simulink model "passivity_based_control"  (R2025a)
settings: Solver=VariableStepAuto  StartTime=0.0  StopTime=115  RelTol=1e-3
values from neighbouring files (symbols this model uses):
  Dxy = 1    [main_passivity_based_control.m]
  Dyaw = -0.8    [main_passivity_based_control.m]
  eta_b_0 = [0 0 0]    [main_passivity_based_control.m]
  eta_b_dot_0 = [0 0 0]    [main_passivity_based_control.m]
  f_e = [Dxy Dxy Dz]    [main_passivity_based_control.m]
  g = 9.81    [main_passivity_based_control.m]
  Ib = diag([1.2416 1.2416 2*1.2416])    [main_passivity_based_control.m]
  K = flip(K)    [main_passivity_based_control.m]
  K_a = 1.25    [main_passivity_based_control.m]
  K_r = 0.5    [main_passivity_based_control.m]
  lin_vel_0 = [0; 0; 0]    [main_passivity_based_control.m]
  mass = 1.2    [main_passivity_based_control.m]
  obstacles_points = [obstacles_points, points]    [main_passivity_based_control.m]
  pos_0 = [x0 y0 z0]    [main_passivity_based_control.m]
  psif = 0    [main_passivity_based_control.m]
  r = 2    [main_passivity_based_control.m]
  rho_0 = 2.0    (= 2)    [main_passivity_based_control.m]
  tau_e = [0 0 Dyaw]    [main_passivity_based_control.m]
  Ts = 0.01    [main_passivity_based_control.m]
  Waypoints = [ 0  20  -6 ... (first row only)    [main_passivity_based_control.m]
undefined symbols (not defined in the file or in its folder): DiscIntNeverNeededParam
libraries: uavsimlib x3, robotcorelib x1, eeGeneralControl x1
settings Model: Creator=emman  LastModifiedBy=emman

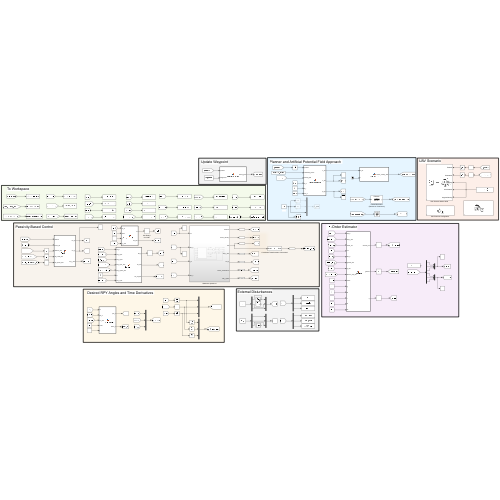
[thumbnail: Simulink's stored preview of the top-level diagram]
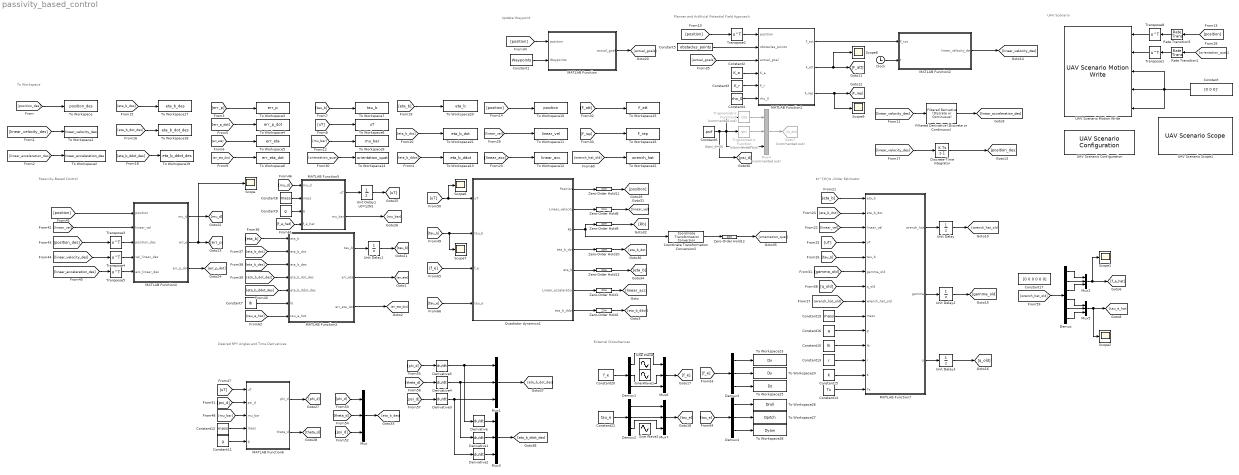
== system passivity_based_control ==
  note: Passivity-Based Control
  note: Desired RPY Angles and Time Derivatives
  note: Update Waypoint
  note: Planner and Artificial Potential Field Approach
  note: UAV Scenario
  note: $\psi_d=0$
  note: To Workspace
  note: $r^{th}$ -Order Estimator
  note: External Disturbances
  Clock : Clock
  Constant : Constant  Value=[0 0 0]'
  Constant1 : Constant  Value=Waypoints
  Constant10 : Constant  Value=Ib
  Constant11 : Constant  Value=g
  Constant12 : Constant  Value=mass
  Constant13 : Constant  Value=r
  Constant14 : Constant  Value=Ts
  Constant15 : Constant  Value=K
  Constant16 : Constant  Value=g
  Constant17 : Constant  Value=[0 0 0 0 0 0]
  Constant19 : Constant  Value=mass
  Constant2 : Constant  Value=K_a
  Constant20 : Constant  Value=f_e
  Constant21 : Constant  Value=tau_e
  Constant3 : Constant  Value=K_r
  Constant4 : Constant  Value=rho_0
  Constant5 : Constant  Value=obstacles_points
  Constant6 : Constant  Value=psif
  Constant7 : Constant  Value=Ib
  Constant8 : Constant  Value=mass
  Constant9 : Constant  Value=g
  Coordinate Transformation Conversion2 : robotcorelib/Coordinate Transformation Conversion  InputRepresentation=Rotation Matrix  InputEulerSequence=ZYX  ShowTrVecInputPort=on  OutputRepresentation=Quaternion  OutputEulerSequence=ZYX  ShowTrVecOutputPort=on  SimulateUsing=Interpreted execution
  Demux : Demux  Outputs=6
  Demux{1..4} (4 alike) : Demux  Outputs=3
  Derivative{,1..5} (6 alike) : Derivative
  Discrete-Time Integrator : DiscreteIntegrator  InitialCondition=pos_0  SampleTime=Ts  ICPrevOutput=DiscIntNeverNeededParam  ICPrevScaledInput=DiscIntNeverNeededParam
  Filtered Derivative (Discrete or Continuous) : eeGeneralControl/Filtered Derivative (Discrete or Continuous)  K=1  T=Ts  B=inf  A=-inf  minRatio=10  init_option=Inherited from block input  x0=0  Ts=-1
      settings: LibrarySourceBlock=|
      | ee_sl_lib/General Control/Filtered Derivative
      | (Discrete or Continuous)
  Goto7 : Goto  Commented=on  GotoTag=xb_des
  MATLAB Function : MATLAB Function  TreatAsAtomicUnit=on
  MATLAB Function1 : MATLAB Function  TreatAsAtomicUnit=on
  MATLAB Function2 : MATLAB Function  TreatAsAtomicUnit=on
  MATLAB Function3 : MATLAB Function  TreatAsAtomicUnit=on
  MATLAB Function4 : MATLAB Function  TreatAsAtomicUnit=on
  MATLAB Function5 : MATLAB Function  TreatAsAtomicUnit=on
  MATLAB Function6 : MATLAB Function  TreatAsAtomicUnit=on
  MATLAB Function7 : MATLAB Function  TreatAsAtomicUnit=on
  Mux{,1..3,5..7} (7 alike) : Mux  Inputs=3
  Mux4 : Mux  Commented=on  Inputs=3
  Quadrotor dynamics1 : Subsystem
  Rate Transition1 : RateTransition  OutPortSampleTime=Ts
  Rate Transition5 : RateTransition  OutPortSampleTime=Ts
  Scope{,1..2,6..9} (7 alike) : Scope
      Scope settings: ActiveDisplayYMinimum=-1  ActiveDisplayYMaximum=1  DataLoggingVariableName=ScopeData3
      Scope1 settings: ActiveDisplayYMinimum=-1  ActiveDisplayYMaximum=1
      Scope2 settings: ActiveDisplayYMinimum=-2.2549630226203039  ActiveDisplayYMaximum=1.6732320406118144
      Scope6 settings: ActiveDisplayYMinimum=11.66748  ActiveDisplayYMaximum=12.03695  DataLoggingVariableName=ScopeData2
      Scope7 settings: ActiveDisplayYMinimum=-0.02035  ActiveDisplayYMaximum=0.02035  DataLoggingVariableName=ScopeData7
      Scope8 settings: ActiveDisplayYMinimum=-10.489441161556352  ActiveDisplayYMaximum=10.433654100091561  DataLoggingVariableName=ScopeData8
      Scope9 settings: ActiveDisplayYMinimum=-1  ActiveDisplayYMaximum=1  DataLoggingVariableName=ScopeData9
  Sine Wave : Sin  Amplitude=Dxy  Frequency=0.5  SampleTime=Ts
  Sine Wave1 : Sin  Amplitude=Dxy  Frequency=0.2  Phase=pi  SampleTime=Ts
  Sine Wave2 : Sin  Amplitude=Dyaw  Frequency=0.1  SampleTime=Ts
  To Workspace : ToWorkspace  VariableName=position_des  SaveFormat=Timeseries  SampleTime=-1
  To Workspace1 : ToWorkspace  VariableName=linear_velocity_des  SaveFormat=Timeseries  SampleTime=-1
  To Workspace10 : ToWorkspace  VariableName=position  SaveFormat=Timeseries  SampleTime=-1
  To Workspace11 : ToWorkspace  VariableName=linear_vel  SaveFormat=Timeseries  SampleTime=-1
  To Workspace12 : ToWorkspace  VariableName=linear_acc  SaveFormat=Timeseries  SampleTime=-1
  To Workspace13 : ToWorkspace  VariableName=eta_b_ddot  SaveFormat=Timeseries  SampleTime=-1
  To Workspace14 : ToWorkspace  VariableName=orientation_quat  SaveFormat=Timeseries  SampleTime=-1
  To Workspace15 : ToWorkspace  VariableName=F_att  SaveFormat=Timeseries  SampleTime=-1
  To Workspace16 : ToWorkspace  VariableName=F_rep  SaveFormat=Timeseries  SampleTime=-1
  To Workspace17 : ToWorkspace  VariableName=eta_b_des  SaveFormat=Timeseries  SampleTime=-1
  To Workspace18 : ToWorkspace  VariableName=eta_b_dot_des  SaveFormat=Timeseries  SampleTime=-1
  To Workspace19 : ToWorkspace  VariableName=eta_b_ddot_des  SaveFormat=Timeseries  SampleTime=-1
  To Workspace2 : ToWorkspace  VariableName=linear_acceleration_des  SaveFormat=Timeseries  SampleTime=-1
  To Workspace20 : ToWorkspace  VariableName=eta_b  SaveFormat=Timeseries  SampleTime=-1
  To Workspace21 : ToWorkspace  VariableName=eta_b_dot  SaveFormat=Timeseries  SampleTime=-1
  To Workspace22 : ToWorkspace  VariableName=wrench_hat  SaveFormat=Timeseries  SampleTime=-1
  To Workspace23 : ToWorkspace  VariableName=Dx  SaveFormat=Timeseries  SampleTime=-1
  To Workspace24 : ToWorkspace  VariableName=Dy  SaveFormat=Timeseries  SampleTime=-1
  To Workspace25 : ToWorkspace  VariableName=Dz  SaveFormat=Timeseries  SampleTime=-1
  To Workspace26 : ToWorkspace  VariableName=Droll  SaveFormat=Timeseries  SampleTime=-1
  To Workspace27 : ToWorkspace  VariableName=Dpitch  SaveFormat=Timeseries  SampleTime=-1
  To Workspace28 : ToWorkspace  VariableName=Dyaw  SaveFormat=Timeseries  SampleTime=-1
  To Workspace3 : ToWorkspace  VariableName=err_p  SaveFormat=Timeseries  SampleTime=-1
  To Workspace4 : ToWorkspace  VariableName=err_p_dot  SaveFormat=Timeseries  SampleTime=-1
  To Workspace5 : ToWorkspace  VariableName=err_eta  SaveFormat=Timeseries  SampleTime=-1
  To Workspace6 : ToWorkspace  VariableName=err_eta_dot  SaveFormat=Timeseries  SampleTime=-1
  To Workspace7 : ToWorkspace  VariableName=tau_b  SaveFormat=Timeseries  SampleTime=-1
  To Workspace8 : ToWorkspace  VariableName=uT  SaveFormat=Timeseries  SampleTime=-1
  To Workspace9 : ToWorkspace  VariableName=mu_bar  SaveFormat=Timeseries  SampleTime=-1
  Transpose{1..5,8} (6 alike) : Math  Operator=transpose
  Trigonometric Function : Trigonometry  Commented=on
  Trigonometric Function1 : Trigonometry  Commented=on  Operator=cos
  UAV Scenario Configuration : uavsimlib/UAV Scenario Configuration  Priority=-1  UAVScenarioObject=Scenario  SampleTime=Ts  UpdateParam=false  SensorMotionBusName='SensorMotionBus'  PlatformMotionBusName='PlatformMotionBus'  ScenarioMotionBusName='ScenarioMotionBus'  ScenarioMotionSignalName='ScenarioMotions'
  UAV Scenario Motion Write : uavsimlib/UAV Scenario Motion Write  Priority=0  PlatName='UAV'  ReferenceFrame=NED
  UAV Scenario Scope1 : uavsimlib/UAV Scenario Scope  Priority=1  SensorNameTable={}  SampleTime=Ts
  Unit Delay : UnitDelay  InitialCondition=zeros(6,1)  SampleTime=Ts  HasFrameUpgradeWarning=on
  Unit Delay1 : UnitDelay  InitialCondition=[0 0 0]'  SampleTime=Ts
  Unit Delay1 u0=12N1 : UnitDelay  InitialCondition=12  SampleTime=Ts
  Unit Delay2 : UnitDelay  InitialCondition=zeros(6,r)  SampleTime=Ts  HasFrameUpgradeWarning=on
  Unit Delay3 : UnitDelay  InitialCondition=zeros(6,1)  SampleTime=Ts  HasFrameUpgradeWarning=on
  Zero-Order Hold{1..2,8..13} (8 alike) : ZeroOrderHold  SampleTime=Ts
  wires:
  [linear_velocity_des] -> To Workspace1/1
  [tau_b] -> To Workspace7/1
  [err_eta] -> To Workspace5/1
  [position_des] -> To Workspace/1
  [linear_acceleration_des] -> To Workspace2/1
  [uT] -> To Workspace8/1
  [mu_bar] -> To Workspace9/1
  [err_p] -> To Workspace3/1
  Constant2/1 -> MATLAB Function1/4(K_a)
  Constant3/1 -> MATLAB Function1/5(K_r)
  Constant4/1 -> MATLAB Function1/6(rho_0)
  MATLAB Function1/1(F_tot) -> MATLAB Function2/1(F_tot)
  Clock/1 -> MATLAB Function2/2(t)
  MATLAB Function1/2(F_att) -> Scope8/1, [F_att]
  Trigonometric Function1/1 -> Mux4/1
  Mux4/1 -> Goto7/1
  Constant6/1 -> [psi_d], Mux4/3, Trigonometric Function/1, Trigonometric Function1/1
  Trigonometric Function/1 -> Mux4/2
  [linear_velocity_des] -> Filtered Derivative (Discrete or Continuous)/1
  [linear_velocity_des] -> Discrete-Time Integrator/1
  Constant/1 -> UAV Scenario Motion Write/5, UAV Scenario Motion Write/3, UAV Scenario Motion Write/4
  Constant5/1 -> MATLAB Function1/2(obstacles_points)
  Rate Transition5/1 -> Transpose8/1
  [position] -> Rate Transition5/1
  Transpose8/1 -> UAV Scenario Motion Write/1
  Rate Transition1/1 -> Transpose1/1
  Transpose1/1 -> UAV Scenario Motion Write/2
  [orientation_quat] -> Rate Transition1/1
  [position] -> To Workspace10/1
  [linear_acc] -> To Workspace12/1
  [linear_vel] -> To Workspace11/1
  [eta_b_ddot] -> To Workspace13/1
  [orientation_quat] -> To Workspace14/1
  [F_rep] -> To Workspace16/1
  [F_att] -> To Workspace15/1
  [position] -> Transpose2/1
  Transpose2/1 -> MATLAB Function1/1(position)
  MATLAB Function1/3(F_rep) -> [F_rep], Scope9/1
  [actual_goals] -> MATLAB Function1/3(actual_goal)
  Constant1/1 -> MATLAB Function/2(Waypoints)
  MATLAB Function/1(actual_goal) -> [actual_goals]
  [position] -> MATLAB Function/1(position)
  [eta_b] -> MATLAB Function3/1(eta_b)
  [eta_b_dot] -> MATLAB Function3/2(eta_b_dot)
  [eta_b_des] -> MATLAB Function3/3(eta_b_des)
  [eta_b_dot_des] -> MATLAB Function3/4(eta_b_dot_des)
  [eta_b_ddot_des] -> MATLAB Function3/5(eta_b_ddot_des)
  Constant7/1 -> MATLAB Function3/6(Ib)
  MATLAB Function3/1(tau_b) -> Unit Delay1/1
  Unit Delay1/1 -> [tau_b]
  [linear_acceleration_des] -> Transpose5/1
  [linear_velocity_des] -> Transpose4/1
  [position_des] -> Transpose3/1
  [linear_vel] -> MATLAB Function4/2(linear_vel)
  [position] -> MATLAB Function4/1(position)
  MATLAB Function4/1(mu_d) -> [mu_d]
  MATLAB Function4/3(err_p_dot) -> [err_p_dot]
  MATLAB Function4/2(err_p) -> Scope/1, [err_p]
  Constant9/1 -> MATLAB Function5/3(g)
  Constant8/1 -> MATLAB Function5/2(mass)
  [mu_d] -> MATLAB Function5/1(mu_d)
  MATLAB Function5/1(uT) -> Unit Delay1 u0=12N1/1
  Unit Delay1 u0=12N1/1 -> [uT]
  MATLAB Function5/2(mu_bar) -> [mu_bar]
  [uT] -> MATLAB Function6/1(uT)
  [mu_bar] -> MATLAB Function6/3(mu_bar)
  Constant12/1 -> MATLAB Function6/4(mass)
  Constant11/1 -> MATLAB Function6/5(g)
  MATLAB Function6/1(phi_d) -> [phi_d]
  MATLAB Function6/2(theta_d) -> [theta_d]
  Quadrotor dynamics1/3(Rb) -> Zero-Order Hold9/1, Coordinate Transformation Conversion2/1
  [tau_b] -> Quadrotor dynamics1/2(tau_b), Scope7/1
  Zero-Order Hold11/1 -> [position]
  Zero-Order Hold12/1 -> [orientation_quat]
  Zero-Order Hold8/1 -> [linear_vel]
  Coordinate Transformation Conversion2/1 -> Zero-Order Hold12/1
  Quadrotor dynamics1/1(Position) -> Zero-Order Hold11/1
  [uT] -> Scope6/1, Quadrotor dynamics1/1(uT)
  Quadrotor dynamics1/2(Linear_velocity) -> Zero-Order Hold8/1
  Zero-Order Hold9/1 -> [Rb]
  Quadrotor dynamics1/4(eta_b_dot) -> Zero-Order Hold10/1
  Quadrotor dynamics1/5(eta_b) -> Zero-Order Hold13/1
  [psi_d] -> MATLAB Function6/2(psi_d)
  [phi_d] -> Mux/1
  [theta_d] -> Mux/2
  [psi_d] -> Mux/3
  Mux/1 -> [eta_b_des]
  [phi_d] -> Derivative5/1
  [theta_d] -> Derivative4/1
  [psi_d] -> Derivative3/1
  Derivative3/1 -> Derivative2/1, Mux1/3
  Derivative4/1 -> Derivative1/1, Mux1/2
  Derivative5/1 -> Derivative/1, Mux1/1
  Mux1/1 -> [eta_b_dot_des]
  Derivative1/1 -> Mux3/2
  Derivative2/1 -> Mux3/3
  Derivative/1 -> Mux3/1
  Mux3/1 -> [eta_b_ddot_des]
  Transpose3/1 -> MATLAB Function4/3(position_des)
  Transpose4/1 -> MATLAB Function4/4(vel_linear_des)
  Transpose5/1 -> MATLAB Function4/5(acc_linear_des)
  MATLAB Function2/1(linear_velocity_des) -> [linear_velocity_des]
  Discrete-Time Integrator/1 -> [position_des]
  Zero-Order Hold10/1 -> [eta_b_dot]
  Zero-Order Hold13/1 -> [eta_b]
  Filtered Derivative (Discrete or Continuous)/1 -> [linear_acceleration_des]
  MATLAB Function3/3(err_eta_dot) -> [err_eta_dot]
  MATLAB Function3/2(err_eta) -> [err_eta]
  Quadrotor dynamics1/6(Linear_acceleration) -> Zero-Order Hold1/1
  Zero-Order Hold1/1 -> [linear_acc]
  Quadrotor dynamics1/7(eta_b_ddot) -> Zero-Order Hold2/1
  Zero-Order Hold2/1 -> [eta_b_ddot]
  [err_p_dot] -> To Workspace4/1
  [err_eta_dot] -> To Workspace6/1
  [eta_b_des] -> To Workspace17/1
  [eta_b_dot_des] -> To Workspace18/1
  [eta_b_ddot_des] -> To Workspace19/1
  [eta_b] -> To Workspace20/1
  [eta_b_dot] -> To Workspace21/1
  [q_old] -> MATLAB Function7/7(q_old)
  [wrench_hat_old] -> MATLAB Function7/8(wrench_hat_old)
  Demux/4 -> Mux5/1
  Demux/5 -> Mux5/2
  Mux2/1 -> Scope1/1, [f_e_hat]
  Demux/6 -> Mux5/3
  [gamma_old] -> MATLAB Function7/6(gamma_old)
  Demux/1 -> Mux2/1
  Unit Delay2/1 -> [gamma_old]
  Demux/2 -> Mux2/2
  MATLAB Function7/3(q) -> Unit Delay3/1
  MATLAB Function7/1(wrench_hat) -> Unit Delay/1
  Constant10/1 -> MATLAB Function7/11(Ib)
  [tau_b] -> MATLAB Function7/5(tau_b)
  [linear_vel] -> MATLAB Function7/3(linear_vel)
  Mux5/1 -> Scope2/1, [tau_e_hat]
  Unit Delay/1 -> [wrench_hat_old]
  MATLAB Function7/2(gamma) -> Unit Delay2/1
  [uT] -> MATLAB Function7/4(uT)
  Constant13/1 -> MATLAB Function7/12(r)
  Constant14/1 -> MATLAB Function7/14(Ts)
  Constant16/1 -> MATLAB Function7/10(g)
  Demux/3 -> Mux2/3
  Constant19/1 -> MATLAB Function7/9(mass)
  Unit Delay3/1 -> [q_old]
  Constant15/1 -> MATLAB Function7/13(K)
  [eta_b] -> MATLAB Function7/1(eta_b)
  [eta_b_dot] -> MATLAB Function7/2(eta_b_dot)
  [wrench_hat_old] -> To Workspace22/1
  [f_e_hat] -> MATLAB Function5/4(f_e_hat)
  [tau_e_hat] -> MATLAB Function3/7(tau_e_hat)
  [f_e] -> Quadrotor dynamics1/3(f_e)
  [tau_e] -> Quadrotor dynamics1/4(tau_e)
  Demux4/2 -> To Workspace27/1
  Demux4/3 -> To Workspace28/1
  Demux3/1 -> To Workspace23/1
  [tau_e] -> Demux4/1
  Demux3/3 -> To Workspace25/1
  [f_e] -> Demux3/1
  Demux4/1 -> To Workspace26/1
  Mux7/1 -> [tau_e]
  Demux2/1 -> Mux7/1
  Demux2/2 -> Mux7/2
  Demux1/3 -> Mux6/3
  Constant21/1 -> Demux2/1
  Constant20/1 -> Demux1/1
  Demux3/2 -> To Workspace24/1
  Mux6/1 -> [f_e]
  Demux2/3 -> Mux7/3
  Demux1/1 -> Mux6/1
  Demux1/2 -> Mux6/2
  [wrench_hat_old] -> Demux/1

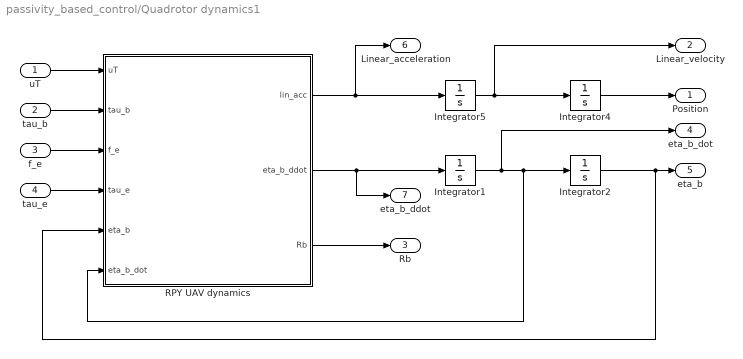
== system passivity_based_control/Quadrotor dynamics1 ==
  uT : Inport
  tau_b : Inport  Port=2
  f_e : Inport  Port=3
  tau_e : Inport  Port=4
  Integrator1 : Integrator  InitialCondition=eta_b_dot_0
  Integrator2 : Integrator  InitialCondition=eta_b_0
  Integrator4 : Integrator  InitialCondition=pos_0
  Integrator5 : Integrator  InitialCondition=lin_vel_0
  RPY UAV dynamics : MATLAB Function  TreatAsAtomicUnit=on
  Position : Outport
  Linear_velocity : Outport  Port=2
  Rb : Outport  Port=3
  eta_b_dot : Outport  Port=4
  eta_b : Outport  Port=5
  Linear_acceleration : Outport  Port=6
  eta_b_ddot : Outport  Port=7
  wires:
  tau_b/1 -> RPY UAV dynamics/2(tau_b)
  uT/1 -> RPY UAV dynamics/1(uT)
  RPY UAV dynamics/3(Rb) -> Rb/1
  RPY UAV dynamics/2(eta_b_ddot) -> eta_b_ddot/1, Integrator1/1
  Integrator5/1 -> Linear_velocity/1, Integrator4/1
  RPY UAV dynamics/1(lin_acc) -> Linear_acceleration/1, Integrator5/1
  Integrator4/1 -> Position/1
  Integrator1/1 -> RPY UAV dynamics/6(eta_b_dot), Integrator2/1, eta_b_dot/1
  Integrator2/1 -> RPY UAV dynamics/5(eta_b), eta_b/1
  f_e/1 -> RPY UAV dynamics/3(f_e)
  tau_e/1 -> RPY UAV dynamics/4(tau_e)

== matlab function passivity_based_control/MATLAB Function5 ==
  data: mu_d input; uT output; mass input; g input; mu_bar output; f_e_hat input
function [uT, mu_bar] = ThrustComputation(mu_d, mass, g, f_e_hat)

%% mu_d Components
% Without Estimator mu_bar = mu_d
mu_bar = mu_d - 1/mass*f_e_hat;

mu_bar_x = mu_bar(1);
mu_bar_y = mu_bar(2);
mu_bar_z = mu_bar(3);

uT = mass*sqrt(mu_bar_x^2 + mu_bar_y^2 + (mu_bar_z - g)^2);

== matlab function passivity_based_control/MATLAB Function6 ==
  data: uT input; phi_d output; psi_d input; mu_bar input; mass input; g input; theta_d output
function [phi_d, theta_d] = AttitudeComputation(uT, psi_d, mu_bar, mass, g)

%% mu_bar Components
mu_bar_x = mu_bar(1);
mu_bar_y = mu_bar(2);
mu_bar_z = mu_bar(3);

%% Desired Roll and Pitch Angles (the Yaw Angle is given by the Planner)
phi_d = asin((mass/uT)*(mu_bar_y*cos(psi_d) - mu_bar_x*sin(psi_d)));
theta_d = atan((mu_bar_x*cos(psi_d) + mu_bar_y*sin(psi_d))/(mu_bar_z - g));

== matlab function passivity_based_control/Quadrotor dynamics1/RPY UAV dynamics ==
  data: uT input size=1; tau_b input size=3; f_e input; tau_e input; lin_acc output size=3; eta_b_ddot output size=3; eta_b input size=3; eta_b_dot input size=3; Rb output size=[3,3]; mass parameter size=1; Ib parameter size=[3,3]
function [lin_acc, eta_b_ddot, Rb] = RPYQuadrotorDynamicModel(uT, tau_b, f_e, tau_e, eta_b, eta_b_dot, mass, Ib)

%% RPY Angles and Time Derivatives
phi = eta_b(1);
theta = eta_b(2);
psi = eta_b(3);

phi_dot = eta_b_dot(1);
theta_dot = eta_b_dot(2);
psi_dot = eta_b_dot(3);

%% Matrices Computation
Q = [1 0 -sin(theta);
    0 cos(phi) cos(theta)*cos(phi);
    0 -sin(phi) cos(theta)*cos(phi)];

S=skew(Q*eta_b_dot);

Q_dot=[0 0 -cos(theta)*eta_b_dot(2);
0 -sin(phi)*phi_dot -sin(theta)*sin(phi)*theta_dot+cos(theta)*cos(phi)*phi_dot;
0 -cos(phi)*phi_dot -sin(theta)*cos(phi)*theta_dot-cos(theta)*sin(phi)*phi_dot];

C = Q'*S*Ib*Q + Q'*Ib*Q_dot;

M = Q'*Ib*Q;


Rb=[cos(theta)*cos(psi) sin(phi)*sin(theta)*cos(psi)-cos(phi)*sin(psi) cos(phi)*sin(theta)*cos(psi)+sin(phi)*sin(psi);
    cos(theta)*sin(psi) sin(phi)*sin(theta)*sin(psi)+cos(phi)*cos(psi) cos(phi)*sin(theta)*sin(psi)-sin(phi)*cos(psi);
-sin(theta) sin(phi)*cos(theta) cos(phi)*cos(theta)];

e_3 = [0 0 1]';

lin_acc = 9.81*e_3 - (uT/mass)*Rb*e_3 + f_e/mass;

eta_b_ddot = inv(M)*(-C*eta_b_dot + Q'*tau_b + tau_e);



end

function S = skew(v)
if(numel(v)~= 1)
S= [0 -v(3) v(2); 
    v(3) 0 -v(1);
    -v(2) v(1) 0];
else
S= zeros(3);
end
end

== matlab function passivity_based_control/MATLAB Function ==
  data: position input; actual_goal output; Waypoints input
function actual_goal = UpdateWaypoint(position, Waypoints)

    persistent idx wp_toll num_wp

    if isempty(idx)
        idx = 1;
        wp_toll = 0.05; % Tolerance Distance
        num_wp = size(Waypoints, 1);
    end

    actual_goal = Waypoints(idx, :);

    % Distance from Current Goal
    dist = norm(position' - actual_goal);

    % Advance to Next Waypoint if close enough
    if dist < wp_toll && idx < num_wp
        idx = idx + 1;
        actual_goal = Waypoints(idx, :);
    end
end

== matlab function passivity_based_control/MATLAB Function7 ==
  data: eta_b input; eta_b_dot input; linear_vel input; uT input; tau_b input; gamma_old input; q_old input; wrench_hat_old input; mass input; g input; Ib input; r input; K input; Ts input; wrench_hat output; gamma output; q output
function [wrench_hat, gamma, q] = Estimator(eta_b, eta_b_dot, linear_vel, uT, tau_b, gamma_old, q_old, wrench_hat_old, mass, g, Ib, r, K, Ts)

    % Estimator considering the Generalised Momentum Vector q
    
    %% RPY Angles and Time Derivatives
    phi = eta_b(1);
    theta = eta_b(2);
    psi = eta_b(3);
    
    phi_dot = eta_b_dot(1);
    theta_dot = eta_b_dot(2);
    psi_dot = eta_b_dot(3);
    
    %% Matrices Computation
    Q = [1 0 -sin(theta);
        0 cos(phi) cos(theta)*cos(phi);
        0 -sin(phi) cos(theta)*cos(phi)];
    
    S=skew(Q*eta_b_dot);
    
    Q_dot=[0 0 -cos(theta)*eta_b_dot(2);
    0 -sin(phi)*phi_dot -sin(theta)*sin(phi)*theta_dot+cos(theta)*cos(phi)*phi_dot;
    0 -cos(phi)*phi_dot -sin(theta)*cos(phi)*theta_dot-cos(theta)*sin(phi)*phi_dot];
    
    C = Q'*S*Ib*Q + Q'*Ib*Q_dot;
    
    M = Q'*Ib*Q;
    
    
    Rb=[cos(theta)*cos(psi) sin(phi)*sin(theta)*cos(psi)-cos(phi)*sin(psi) cos(phi)*sin(theta)*cos(psi)+sin(phi)*sin(psi);
        cos(theta)*sin(psi) sin(phi)*sin(theta)*sin(psi)+cos(phi)*cos(psi) cos(phi)*sin(theta)*sin(psi)-sin(phi)*cos(psi);
    -sin(theta) sin(phi)*cos(theta) cos(phi)*cos(theta)];
    
    e_3 = [0 0 1]';


    q = [mass*eye(3) zeros(3,3); zeros(3,3) M] * [linear_vel; eta_b_dot];

    gamma = gamma_old;
  
    % Gamma 1 Computation
    gamma(:,1) = gamma_old(:,1) + K(1)*((q - q_old) - Ts*[mass*g*e_3 - uT*Rb*e_3; C'*eta_b_dot + Q'*tau_b] - Ts*wrench_hat_old);
    
    % Gamma Computation
    for j = 2:r
        gamma(:,j) = gamma_old(:,j) + K(j)*Ts*(-wrench_hat_old + gamma_old(:,j-1));
    end
      
    % Estimation Update
    wrench_hat = gamma(:,r);



end



function S = skew(v)
if(numel(v)~= 1)
S= [0 -v(3) v(2); 
    v(3) 0 -v(1);
    -v(2) v(1) 0];
else
S= zeros(3);
end
end

function v = wedge(S)
v1 = S(3,2);
v2 = S(1,3);
v3 = S(2,1);
v = [v1 v2 v3]';
end

== matlab function passivity_based_control/MATLAB Function1 ==
  data: position input; F_tot output; obstacles_points input; actual_goal input; K_a input; K_r input; rho_0 input; F_att output; F_rep output
function [F_tot, F_att, F_rep] = ForceComputation(position, obstacles_points, actual_goal, K_a, K_r, rho_0)
% Computes the Total Force (Attractive + Repulsive) for APF (Artificial Potential Field Algorithm)
%
% Inputs:
%   position         - 1x3 UAV Current Position [x, y, z]
%   obstacles_points - 3xN Matrix: each Column is an Obstacle Point [x; y; z] (Different Frame)
%   actual_goal      - 1x3 Actual Goal Position [x, y, z]
%   K_a              - Attractive Gain
%   K_r              - Repulsive Gain
%   rho_0            - Limit Distance of th Potential Field Influence.
%
% Outputs:
%   F_tot            - 1x3 Total Force
%   F_att            - 1x3 Attractive Force
%   F_rep            - 1x3 Repulsive Force


    %% Attractive Force
    % Vector from Current Position to Goal
    e_pos = actual_goal - position;

    if norm(e_pos) < 1
        F_att = K_a * e_pos;
    else
        F_att = K_a * e_pos / norm(e_pos);  % Normalization if too far
    end

    %% Repulsive Force (computed from all obstacle points)
    F_rep = zeros(1, 3);  % Initialize total repulsive force vector

    for i = 1:size(obstacles_points, 2)
        obs_point = obstacles_points(:, i)';  % Extract Obstacles Points [1x3]

        % Compute Distance Vectors (Different Frame between Obstacles and UAV)
        dx = position(1) - obs_point(2);
        dy = position(2) - obs_point(1);
        dz = position(3) - obs_point(3);

        rho = sqrt(dx^2 + dy^2 + dz^2);   % Euclidean Distance 

        
        if rho <= rho_0 && rho > 0
            Gradient = [dx, dy, dz] / rho;  % Gradient (Unit Vector)
            Repulsion = K_r * (1/rho - 1/rho_0) / rho^2 * Gradient;
            F_rep = F_rep + Repulsion;  % Total Repulsive Force
        end
    end

    %% Total Force = Attractive Force + Repulsive Force
    F_tot = F_att + F_rep;
end

== matlab function passivity_based_control/MATLAB Function2 ==
  settings: updateMethod=DISCRETE
  data: F_tot input; t input; linear_velocity_des output
function linear_velocity_des = FilteredVelocity(F_tot, t)
%   This Function apply an Exponential Moving Average Filter to input Total Force Vector
%   It returns the filtered Velocity Vector based on the Input Force Vector F_tot
%   and the Current Time t (for alpha).
%
%   Inputs:
%       F_tot - 1x3 Vector, Total Force Input (from APF Algorithm)
%       t     - Scalar, Current Time (seconds) to compute alpha
%
%   Output:
%       linear_velocity_des - 1x3 Vector, Filtered (Desired) Velocity

% Explanation:
%   In Potential Field Methods, the Output Force Vector represents the direction 
%   and magnitude of "pull" or "push" on the UAV.
%   By applying an Exponential Moving Average Filter to this Force, we can
%   generate a Smoother Velocity Command (linear_velocity_des) that avoids abrupt changes.
%
%   This approach assumes a Proportional relationship between Force and Velocity,
%   effectively treating the Filtered Force as a Desired Velocity Signal.

    % Persistent Variable to store Previous Filtered Velocity
    persistent linear_vel_prev

    if isempty(linear_vel_prev)
        linear_vel_prev = [0 0 0]; % Initialize on First Call
    end

    % Calculate Dynamic Smoothing Factor alpha based on time t
    alpha = alphaComputation(t);

    % Apply Exponential Moving Average Filter
    linear_velocity_des = (1 - alpha) * linear_vel_prev + alpha * F_tot;

    % Update Persistent Variable for Next Iteration
    linear_vel_prev = linear_velocity_des;
end


function alpha = alphaComputation(t)
%   This second function computes alpha for EMA filter adapting over time
%   It returns a Smoothing Factor alpha that increases quadratically
%   from a small initial value up to a final cap.

    alpha_initial = 5e-7; % Initial very small alpha
    alpha_final = 0.005;  % Max alpha value
    % Quadratic increase of alpha over time (example)
    alpha = alpha_initial * (100 * t / 2)^2;

    % Clamp alpha between Initial and Final Values
    alpha = max(min(alpha, alpha_final), alpha_initial);
end

== matlab function passivity_based_control/MATLAB Function3 ==
  data: eta_b input; tau_b output; eta_b_dot input; eta_b_des input; eta_b_dot_des input; eta_b_ddot_des input; Ib input; err_eta output; err_eta_dot output; tau_e_hat input
function [tau_b, err_eta, err_eta_dot]  = InnerLoop(eta_b, eta_b_dot, eta_b_des, eta_b_dot_des, eta_b_ddot_des, Ib, tau_e_hat)

%% RPY Angles and Time Derivatives
phi = eta_b(1);
theta = eta_b(2);
psi = eta_b(3);

phi_dot = eta_b_dot(1);
theta_dot = eta_b_dot(2);
psi_dot = eta_b_dot(3);

%% Parameters
sigma = 20;
D0 = 15*eye(3);
K0 = sigma*D0;
ni = 10;

%% Matrices Computation
Q = [1 0 -sin(theta);
    0 cos(phi) cos(theta)*cos(phi);
    0 -sin(phi) cos(theta)*cos(phi)];

S = skew(Q*eta_b_dot);

Q_dot = [0 0 -cos(theta)*eta_b_dot(2);
0 -sin(phi)*phi_dot -sin(theta)*sin(phi)*theta_dot+cos(theta)*cos(phi)*phi_dot;
0 -cos(phi)*phi_dot -sin(theta)*cos(phi)*theta_dot-cos(theta)*sin(phi)*phi_dot];

C = Q'*S*Ib*Q + Q'*Ib*Q_dot;

M = Q'*Ib*Q;

%% Reference Quantities
err_eta = eta_b - eta_b_des;
err_eta_dot = eta_b_dot - eta_b_dot_des;

eta_r_dot = eta_b_dot_des - sigma*err_eta;
eta_r_ddot = eta_b_ddot_des - ni*err_eta_dot;

v_eta = err_eta_dot + sigma*err_eta;

%% Passivity-Based Control for the Inner (Angular) Loop
tau_b = inv(Q)'*(M*eta_r_ddot + C*eta_r_dot - tau_e_hat -D0*v_eta - K0*err_eta);

end


%% Functions
function S = skew(v)
if(numel(v)~= 1)
S= [0 -v(3) v(2); 
    v(3) 0 -v(1);
    -v(2) v(1) 0];
else
S= zeros(3);
end
end

function v = wedge(S)
v1 = S(3,2);
v2 = S(1,3);
v3 = S(2,1);
v = [v1 v2 v3]';
end

== matlab function passivity_based_control/MATLAB Function4 ==
  data: position input; mu_d output; linear_vel input; position_des input; vel_linear_des input; acc_linear_des input; err_p output; err_p_dot output
function [mu_d, err_p, err_p_dot] = PositionPD(position, linear_vel, position_des, vel_linear_des, acc_linear_des)

%% Errors
err_p = position - position_des;
err_p_dot = linear_vel-vel_linear_des;

%% Gains
K_P = 10*eye(3);
K_D = 0.5*eye(3);

%% Input
mu_d = -K_P*err_p - K_D*err_p_dot + acc_linear_des;

end
